simulink model "durumi2_comp_lin_nonlin_lon"  (R2022a)
settings: Solver=ode4  StartTime=0.0  StopTime=50  FixedStep=0.01  RelTol=1e-5  EnableMultiTasking=on
values from neighbouring files (symbols this model uses):
  A_lon = A([ku kw kq ktheta], [ku kw kq ktheta])    [cal_linearize_durumi2.m]
  B_lon = B([ku kw kq ktheta], [kde kdp])    [cal_linearize_durumi2.m]
  C_lon = eye(length(A_lon))    [sim_durumi2_lin_nonlin_lon.m]
  D_lon = B_lon*0    [sim_durumi2_lin_nonlin_lon.m]
  u_de = 2    [sim_durumi2_lin_nonlin.m]    (also in sim_durumi2_lin_nonlin_lon.m)
  u_th = 0.1    [sim_durumi2_lin_nonlin.m]    (also in sim_durumi2_lin_nonlin_lon.m)
undefined symbols (not defined in the file or in its folder): sigbuilder_block, u0
libraries: simulink_extras x3
settings Model: Creator=김응태  LastModifiedBy=USer
settings DataIOCC: SaveFormat=Array  SignalLoggingSaveFormat=ModelDataLogs  ReturnWorkspaceOutputs=off  SignalLoggingName=sigsOut
settings OptimizationCC: BooleanDataType=off
settings DebuggingCC: SaveWithParameterizedLinksMsg=none  UnderspecifiedInitializationDetection=Classic  MergeDetectMultiDrivingBlocksExec=none  SignalResolutionControl=TryResolveAllWithWarning  MultiTaskDSMMsg=warning  MultiTaskCondExecSysMsg=none  UnconnectedInputMsg=warning  UnconnectedOutputMsg=warning  UnconnectedLineMsg=warning
settings HardwareCC: ProdBitPerPointer=32  ProdBitPerSizeT=32  ProdBitPerPtrDiffT=32  ProdLargestAtomicFloat=None  ProdIntDivRoundTo=Undefined  ProdEndianess=Unspecified  ProdWordSize=32  ProdHWDeviceType=32-bit Generic  TargetUnknown=on
settings ModelReferenceCC: PropagateSignalLabelsOutOfModel=off
settings GRTTargetCC: CombineOutputUpdateFcns=off  GRTInterface=on
settings ConfigComp: CovMetricSettings=dw  CovSaveCumulativeToWorkspaceVar=on  CovSaveSingleToWorkspaceVar=on

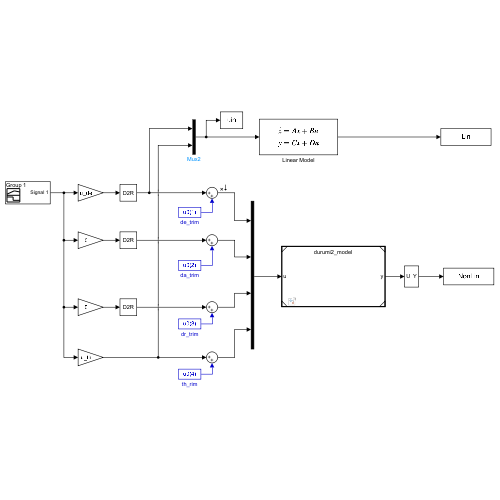
[thumbnail: Simulink's stored preview of the top-level diagram]
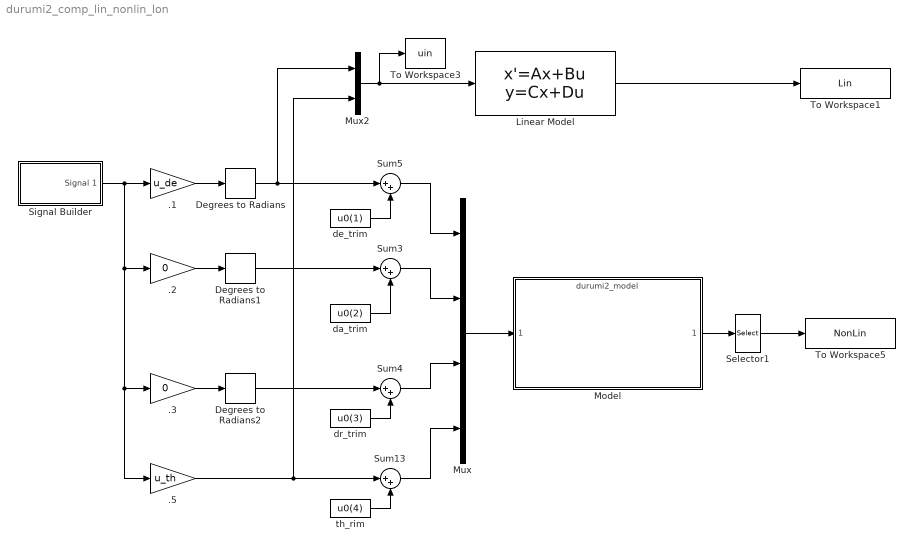
== system durumi2_comp_lin_nonlin_lon ==
  .1 : Gain  Gain=u_de  OutDataTypeStr=Inherit: Same as input  ParamDataTypeStr=Inherit: Same as input
  .2 : Gain  Gain=0  OutDataTypeStr=Inherit: Same as input  ParamDataTypeStr=Inherit: Same as input
  .3 : Gain  Gain=0  OutDataTypeStr=Inherit: Same as input  ParamDataTypeStr=Inherit: Same as input
  .5 : Gain  Gain=u_th  OutDataTypeStr=Inherit: Same as input  ParamDataTypeStr=Inherit: Same as input
  Degrees to Radians : simulink_extras/Transformations/Degrees to Radians
  Degrees to Radians1 : simulink_extras/Transformations/Degrees to Radians
  Degrees to Radians2 : simulink_extras/Transformations/Degrees to Radians
  Linear Model : StateSpace  A=A_lon  B=B_lon  C=C_lon  D=D_lon  InitialCondition=[0 0 0 0]'
  Model : ModelReference  ModelNameDialog=durumi2_model.slx  SimulationMode=Normal  ModelReferenceVersion=1.76
  Mux : Mux
  Mux2 : Mux  Inputs=2
  Selector1 : Selector  InputPortWidth=12  IndexOptions=Index vector (dialog)  Indices=[1 3 5 8]  OutputSizes=1
  Signal Builder : Subsystem  Tag=STV Subsys  LoadFcn=sigbuilder_block('load');  StartFcn=sigbuilder_block('start');  StopFcn=sigbuilder_block('stop');  ClipboardFcn=sigbuilder_block('clipboard');  mask(Sigbuilder block){tuvar=[0:10]}
      mask help: Simulink:masks:SigbuilderBlock_MD
      mask init:
      | if ~strcmp(get_param(bdroot(gcbh),'SimulationStatus'),'stopped') tuvar = sigbuilder_block('maskInit'); end
      settings: CopyFcn=sigbuilder_block('copy');  DeleteFcn=sigbuilder_block('delete');  ModelCloseFcn=sigbuilder_block('modelClose');  PreSaveFcn=sigbuilder_block('preSave');  PauseFcn=sigbuilder_block('pause');  ContinueFcn=sigbuilder_block('continue');  NameChangeFcn=sigbuilder_block('namechange');  OpenFcn=sigbuilder_block('open',[437.6 199.2 550.4 400 ]);  CloseFcn=sigbuilder_block('close');
      mask Display: plot(0, 0, 100, 100,[2, 2, 32, 32, 2], [68, 8, 8, 68, 68],[32, 2], [38, 38], [32, 19, 2],[53, 60, 44], [32, 17, 17, 2],[16, 16, 31, 31]);txt = getActiveGroup(gcbh);text(2, 100, txt,'verticalAlignment', 'top');
  Sum{3..5,13} (4 alike) : Sum  Inputs=|++  InputSameDT=on  OutDataTypeStr=Inherit: Same as first input
  To Workspace1 : ToWorkspace  VariableName=Lin  SampleTime=-1
  To Workspace3 : ToWorkspace  VariableName=uin  SampleTime=-1
  To Workspace5 : ToWorkspace  VariableName=NonLin  SampleTime=-1
  da_trim : Constant  Value=u0(2)  VectorParams1D=off
  de_trim : Constant  Value=u0(1)  VectorParams1D=off
  dr_trim : Constant  Value=u0(3)  VectorParams1D=off
  th_rim : Constant  Value=u0(4)  VectorParams1D=off
  wires:
  Sum3/1 -> Mux/2
  Sum13/1 -> Mux/4
  da_trim/1 -> Sum3/2
  th_rim/1 -> Sum13/2
  dr_trim/1 -> Sum4/2
  de_trim/1 -> Sum5/2
  Sum4/1 -> Mux/3
  Sum5/1 -> Mux/1
  Mux/1 -> Model/1
  Signal Builder/1(Signal 1) -> .2/1, .3/1, .5/1, .1/1
  Selector1/1 -> To Workspace5/1
  Model/1 -> Selector1/1
  Degrees to Radians2/1 -> Sum4/1
  Degrees to Radians1/1 -> Sum3/1
  .1/1 -> Degrees to Radians/1
  .2/1 -> Degrees to Radians1/1
  .3/1 -> Degrees to Radians2/1
  Linear Model/1 -> To Workspace1/1
  Mux2/1 -> To Workspace3/1, Linear Model/1
  .5/1 -> Sum13/1, Mux2/2
  Degrees to Radians/1 -> Mux2/1, Sum5/1

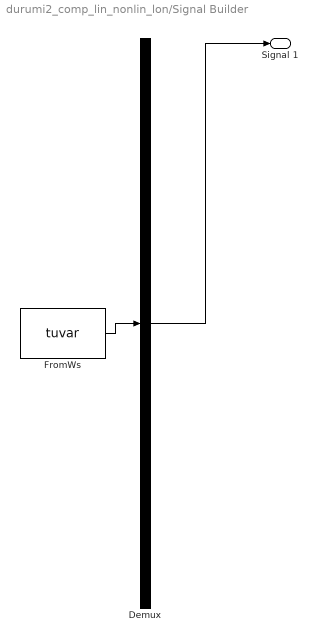
== system durumi2_comp_lin_nonlin_lon/Signal Builder ==
  Demux : Demux  Tag=STV Demux  Outputs=1
      settings: DisplayOption=none
  FromWs : FromWorkspace  Tag=STV FromWs  VariableName=tuvar
      SigBuilderData=|
      | common.afterFinalStr = 'Extrapolate'
      | common.sampleTime = 0
      | dataSet.timeRange = [0 10]
      | dataSet.name = 'Group 1'
      | sbobj.Groups.Name = 'Group 1'
      | sbobj.Groups.Signals.Name = 'Signal 1'
      | sbobj.Groups.Signals.XData = [0 4 4 5 5 6 6 6.96 6.96 10]
      | sbobj.Groups.Signals.YData = [0 0 1 1 0 0 -1 -1 0 0]
      | sbobj.Groups.TimeRange = [0 10]
  Signal 1 : Outport  Tag=STV Outport
  wires:
  FromWs/1 -> Demux/1
  Demux/1 -> Signal 1/1
